simulink model "control_per_channel"  (R2024a)
settings: Solver=FixedStepAuto  StartTime=0.0  StopTime=5  FixedStep=0.002  RelTol=1e-3  EnableMultiTasking=on
settings Model: ExtModeTrigDuration=2  Creator=Jesper  LastModifiedBy=20215368
settings SolverCC: PositivePriorityOrder=on
settings OptimizationCC: EnhancedBackFolding=on  PassReuseOutputArgsAs=Individual arguments  ZeroExternalMemoryAtStartup=off  ZeroInternalMemoryAtStartup=off  MaxStackSize=64  OptimizeBlockOrder=speed  DifferentSizesBufferReuse=on  OptimizationCustomize=off  EfficientTunableParamExpr=on
settings DebuggingCC: ParameterTunabilityLossMsg=error
settings HardwareCC: ProdBitPerPointer=32  ProdBitPerSizeT=32  ProdBitPerPtrDiffT=32  ProdLargestAtomicInteger=Long  ProdLargestAtomicFloat=Double  ProdWordSize=32  ProdLongLongMode=on  ProdHWDeviceType=ARM Compatible->ARM Cortex  UseEmbeddedCoderFeatures=off
settings RTWCC: Description=Embedded Coder  SystemTargetFile=ert.tlc  HardwareBoard=Raspberry Pi  TLCOptions="-aInlineSetEventsForThisBaseRateFcn=TLC_FALSE -aSuppressMultiTaskScheduler=TLC_FALSE  -aRateBasedStepFcn=0"  TemplateMakefile=ert_default_tmf  Toolchain=GNU GCC Embedded Linux  BuildConfiguration=Debug
settings CodeAppCC: ForceParamTrailComments=on  IgnoreCustomStorageClasses=off  OperatorAnnotations=on  SimulinkDataObjDesc=on  SFDataObjDesc=on  InsertBlockDesc=on
settings ERTTargetCC: SupportNonInlinedSFcns=on  SupportVariableSizeSignals=on  ExtModeTransport=2  ExtModeStaticAlloc=on  ExtModeMexFile=ext_xcp  ExtModeIntrfLevel=Level2 - Open

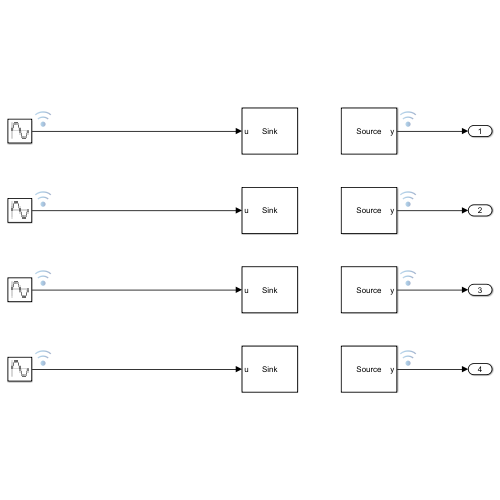
[thumbnail: Simulink's stored preview of the top-level diagram]
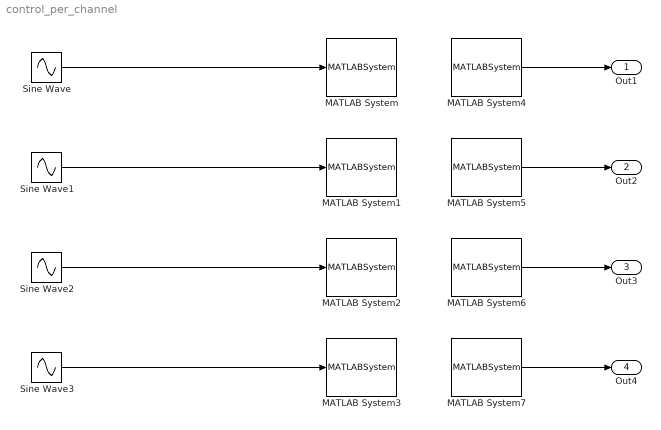
== system control_per_channel ==
  MATLAB System : MATLABSystem  System=Veab_output  i2cbus=1  channel=1  resolution=0.002578125
      mask Type: Veab_output
      mask Display:
      | disp('Sink');
      | port_label('input',1,'u');
  MATLAB System1 : MATLABSystem  System=Veab_output  i2cbus=1  channel=2  resolution=0.002578125
      mask Type: Veab_output
      mask Display:
      | disp('Sink');
      | port_label('input',1,'u');
  MATLAB System2 : MATLABSystem  System=Veab_output  i2cbus=1  channel=3  resolution=0.002578125
      mask Type: Veab_output
      mask Display:
      | disp('Sink');
      | port_label('input',1,'u');
  MATLAB System3 : MATLABSystem  System=Veab_output  i2cbus=1  channel=4  resolution=0.002578125
      mask Type: Veab_output
      mask Display:
      | disp('Sink');
      | port_label('input',1,'u');
  MATLAB System4 : MATLABSystem  System=Veab_input  i2cbus=1  channel=1  resolution=0.002578125  SampleTime=0.002
      mask Type: Veab_input
      mask Display:
      | disp('Source');
      | port_label('output',1,'y');
  MATLAB System5 : MATLABSystem  System=Veab_input  i2cbus=1  channel=2  resolution=0.002578125  SampleTime=0.002
      mask Type: Veab_input
      mask Display:
      | disp('Source');
      | port_label('output',1,'y');
  MATLAB System6 : MATLABSystem  System=Veab_input  i2cbus=1  channel=3  resolution=0.002578125  SampleTime=0.002
      mask Type: Veab_input
      mask Display:
      | disp('Source');
      | port_label('output',1,'y');
  MATLAB System7 : MATLABSystem  System=Veab_input  i2cbus=1  channel=4  resolution=0.002578125  SampleTime=0.002
      mask Type: Veab_input
      mask Display:
      | disp('Source');
      | port_label('output',1,'y');
  Sine Wave : Sin  Amplitude=5  Bias=5  SampleTime=0
  Sine Wave1 : Sin  Amplitude=5  Bias=5  Frequency=2  SampleTime=0
  Sine Wave2 : Sin  Amplitude=5  Bias=5  Frequency=4  SampleTime=0
  Sine Wave3 : Sin  Amplitude=5  Bias=5  Frequency=8  SampleTime=0
  Out1 : Outport
  Out2 : Outport  Port=2
  Out3 : Outport  Port=3
  Out4 : Outport  Port=4
  wires:
  Sine Wave/1 -> MATLAB System/1
  Sine Wave1/1 -> MATLAB System1/1
  Sine Wave2/1 -> MATLAB System2/1
  Sine Wave3/1 -> MATLAB System3/1
  MATLAB System7/1 -> Out4/1
  MATLAB System6/1 -> Out3/1
  MATLAB System5/1 -> Out2/1
  MATLAB System4/1 -> Out1/1
